simulink model "improved_z_source_inverterwithpv"  (Simulink 8.1)
settings: Solver=ode45  StartTime=0.0  StopTime=0.1  MaxStep=1e-6  RelTol=1e-3
libraries: powerlib x128, powerlib_extras x3, simulink x1
settings Model: Creator=Kashif  LastModifiedBy=Rama Krishna Reddy
settings DataIOCC: InspectSignalLogs=on
settings DebuggingCC: SaveWithParameterizedLinksMsg=none  StrictBusMsg=Warning

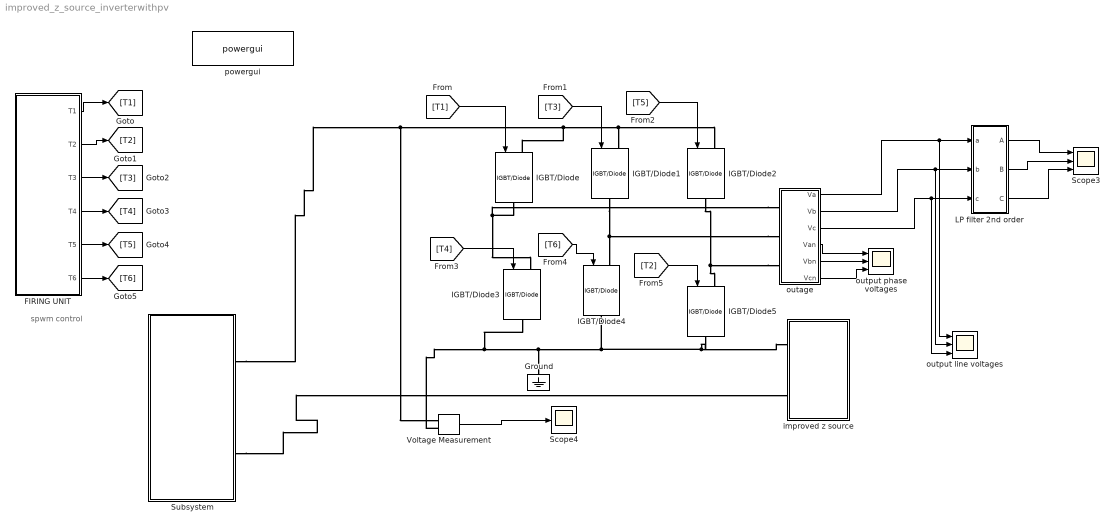
== system improved_z_source_inverterwithpv ==
  note: spwm control
  FIRING UNIT : Subsystem
  Ground : powerlib/Elements/Ground  LConnTagsString=a
  IGBT/Diode{,1..5} (6 alike) : powerlib/Power Electronics/IGBT//Diode  Ron=1e-3  Rs=1e5  Cs=inf  Measurements=off
  LP filter 2nd order : Subsystem  mask{cutoff_frequency=100, damping_factor=0.707}
      mask prompts: cutoff_frequency "Cut off frequency"; damping_factor "Damping Factor"
  Scope3 : Scope  NumInputPorts=3
      settings: TickLabels=on  YMin=-400~-400~-400  YMax=400~400~400  SaveName=Filtered_voltages  MaxDataPoints=5000000  SampleInput=on  SampleTime=5e-6
  Scope4 : Scope
      settings: YMin=362.27  YMax=362.37  SaveName=Neutral_voltages1  MaxDataPoints=5000000  SampleInput=on  SampleTime=5e-6
  Subsystem : Subsystem
  Voltage Measurement : powerlib/Measurements/Voltage Measurement  PhasorSimulation=off  OutputType=Complex  PSBequivalent=0
  improved z source : Subsystem
  outage : Subsystem
  output line voltages : Scope  NumInputPorts=3
      settings: YMin=-5~-5~-5  YMax=5~5~5  SaveName=Line_voltages  MaxDataPoints=5000000  SampleInput=on  SampleTime=5e-6
  output phase voltages : Scope  NumInputPorts=3
      settings: YMin=-250~-250~-250  YMax=250~250~250  SaveName=Neutral_voltages  MaxDataPoints=5000000  SampleInput=on  SampleTime=5e-6
  powergui : powerlib/powergui  Priority=1  SimulationMode=Discrete  SolverType=Tustin  SampleTime=5e-6  frequency=60  SPID=off  DisableSnubberDevices=off  DisableRonSwitches=off  DisableVfSwitches=off  SwTol=0  Interpol=off  DisplayEquations=off  frequencyindice=0  Pbase=100e6  ErrMax=1e-4  Iterations=50  UnitsV=kV  UnitsW=MW  FunctionMessages=off  echomessages=off  HookPort=off  EnableUseOfTLC=off  x0status=blocks  RestoreLinks=warning  ResistiveCurrentMeasurement=off  Frange=[0:2:500]  Ylog=off  Xlog=on  ShowGrid=off  save=off  variable=ZData  structure=Neutral_voltages  ZoomFFT=off  StartTime=0.04  cycles=3  DisplayStyle=2  fundamental=50  FreqAxis=off  MaxFrequency=1000  frequencyindicesteady=1  RmsSteady=1  display=off  Ts=0  methode=off
  wires:
  outage/2(Vb) -> output line voltages/2, LP filter 2nd order/2(b)
  outage/3(Vc) -> output line voltages/3, LP filter 2nd order/3(c)
  outage/4(Van) -> output phase voltages/1
  outage/5(Vbn) -> output phase voltages/2
  outage/6(Vcn) -> output phase voltages/3
  [T3] -> IGBT/Diode1/1
  [T5] -> IGBT/Diode2/1
  [T4] -> IGBT/Diode3/1
  [T6] -> IGBT/Diode4/1
  [T2] -> IGBT/Diode5/1
  [T1] -> IGBT/Diode/1
  FIRING UNIT/1(T1) -> [T1]
  FIRING UNIT/2(T2) -> [T2]
  FIRING UNIT/3(T3) -> [T3]
  FIRING UNIT/4(T4) -> [T4]
  FIRING UNIT/5(T5) -> [T5]
  FIRING UNIT/6(T6) -> [T6]
  outage/1(Va) -> output line voltages/1, LP filter 2nd order/1(a)
  LP filter 2nd order/3(C) -> Scope3/3
  LP filter 2nd order/2(B) -> Scope3/2
  LP filter 2nd order/1(A) -> Scope3/1
  Voltage Measurement/1 -> Scope4/1
  connections:
  outage/LConn1 -- IGBT/Diode3/LConn1 -- IGBT/Diode/RConn1
  outage/LConn2 -- IGBT/Diode4/LConn1 -- IGBT/Diode1/RConn1
  outage/LConn3 -- IGBT/Diode2/RConn1 -- IGBT/Diode5/LConn1
  Voltage Measurement/LConn2 -- IGBT/Diode4/RConn1 -- IGBT/Diode5/RConn1 -- improved z source/LConn1 -- Ground/LConn1 -- IGBT/Diode3/RConn1
  Subsystem/RConn1 -- IGBT/Diode1/LConn1 -- IGBT/Diode2/LConn1 -- IGBT/Diode/LConn1 -- Voltage Measurement/LConn1
  Subsystem/RConn2 -- improved z source/LConn2

== system improved_z_source_inverterwithpv/FIRING UNIT ==
  note: 3-phase input
  Subsystem2 : Subsystem
  Subsystem3 : Subsystem
  T1 : Outport
  T2 : Outport  Port=2
  T3 : Outport  Port=3
  T4 : Outport  Port=4
  T5 : Outport  Port=5
  T6 : Outport  Port=6
  wires:
  Subsystem2/3(SinewaveC) -> Subsystem3/3(In3)
  Subsystem3/1(A1) -> T1/1
  Subsystem3/2(C2) -> T2/1
  Subsystem3/3(B1) -> T3/1
  Subsystem3/4(A2) -> T4/1
  Subsystem3/5(B2) -> T6/1
  Subsystem3/6(C1) -> T5/1
  Subsystem2/1(SinewaveA) -> Subsystem3/1(In1)
  Subsystem2/2(SinewaveB) -> Subsystem3/2(In2)

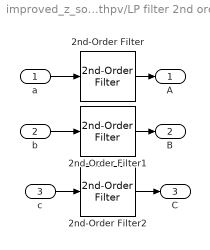
== system improved_z_source_inverterwithpv/LP filter 2nd order ==
  a : Inport
  b : Inport  Port=2
  c : Inport  Port=3
  2nd-Order Filter : powerlib_extras/Control  Blocks/2nd-Order Filter  FilterType=Lowpass  Fo=cutoff_frequency  Zeta=damping_factor  Initialize=off  Vac_Init=[1 45 60]  Vdc_Init=-0.5  PlotResponse=off  param1=[1 500 1]
  2nd-Order Filter1 : powerlib_extras/Control  Blocks/2nd-Order Filter  FilterType=Lowpass  Fo=cutoff_frequency  Zeta=damping_factor  Initialize=off  Vac_Init=[1 45 60]  Vdc_Init=-0.5  PlotResponse=off  param1=[1 500 1]
  2nd-Order Filter2 : powerlib_extras/Control  Blocks/2nd-Order Filter  FilterType=Lowpass  Fo=cutoff_frequency  Zeta=damping_factor  Initialize=off  Vac_Init=[1 45 60]  Vdc_Init=-0.5  PlotResponse=off  param1=[1 500 1]
  A : Outport
  B : Outport  Port=2
  C : Outport  Port=3
  wires:
  a/1 -> 2nd-Order Filter/1
  2nd-Order Filter/1 -> A/1
  b/1 -> 2nd-Order Filter1/1
  2nd-Order Filter1/1 -> B/1
  c/1 -> 2nd-Order Filter2/1
  2nd-Order Filter2/1 -> C/1

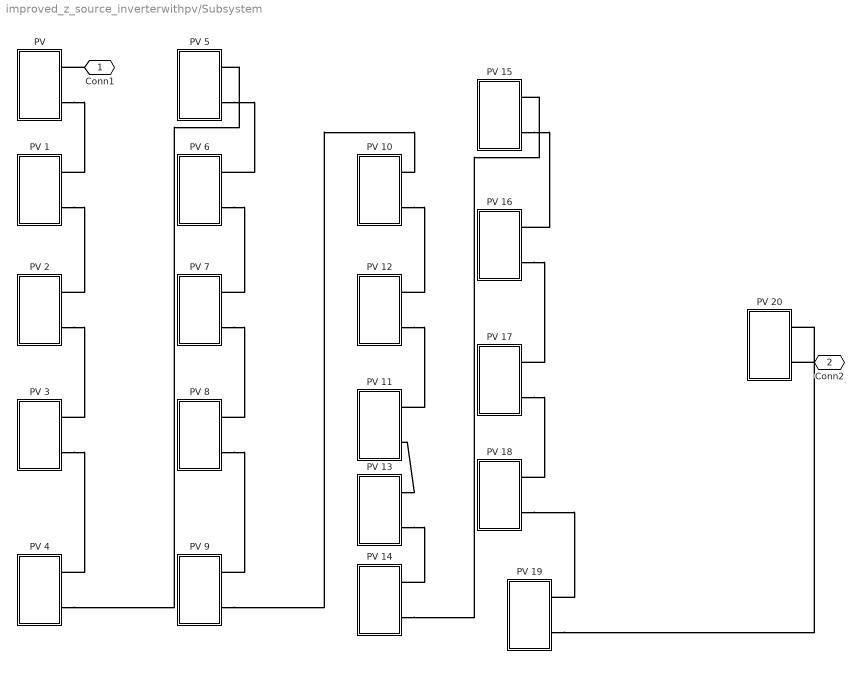
== system improved_z_source_inverterwithpv/Subsystem ==
  "PV " : Subsystem
  PV 1 : Subsystem
  PV 10 : Subsystem
  PV 11 : Subsystem
  PV 12 : Subsystem
  PV 13 : Subsystem
  PV 14 : Subsystem
  PV 15 : Subsystem
  PV 16 : Subsystem
  PV 17 : Subsystem
  PV 18 : Subsystem
  PV 19 : Subsystem
  PV 2 : Subsystem
  PV 20 : Subsystem
  PV 3 : Subsystem
  PV 4 : Subsystem
  PV 5 : Subsystem
  PV 6 : Subsystem
  PV 7 : Subsystem
  PV 8 : Subsystem
  PV 9 : Subsystem
  Conn1 : PMIOPort  Port=1  Side=Right
  Conn2 : PMIOPort  Port=2  Side=Right
  connections:
  "PV "/RConn2 -- PV 1/RConn1
  PV 1/RConn2 -- PV 2/RConn1
  PV 9/RConn2 -- PV 10/RConn1
  PV 10/RConn2 -- PV 12/RConn1
  PV 12/RConn2 -- PV 11/RConn1
  PV 13/RConn1 -- PV 11/RConn2
  PV 13/RConn2 -- PV 14/RConn1
  PV 14/RConn2 -- PV 15/RConn1
  PV 15/RConn2 -- PV 16/RConn1
  PV 16/RConn2 -- PV 17/RConn1
  PV 17/RConn2 -- PV 18/RConn1
  PV 18/RConn2 -- PV 19/RConn1
  PV 19/RConn2 -- PV 20/RConn1
  PV 2/RConn2 -- PV 3/RConn1
  PV 3/RConn2 -- PV 4/RConn1
  PV 4/RConn2 -- PV 5/RConn1
  PV 5/RConn2 -- PV 6/RConn1
  PV 6/RConn2 -- PV 7/RConn1
  PV 7/RConn2 -- PV 8/RConn1
  PV 8/RConn2 -- PV 9/RConn1
  Conn1/RConn1 -- "PV "/RConn1
  Conn2/RConn1 -- PV 20/RConn2

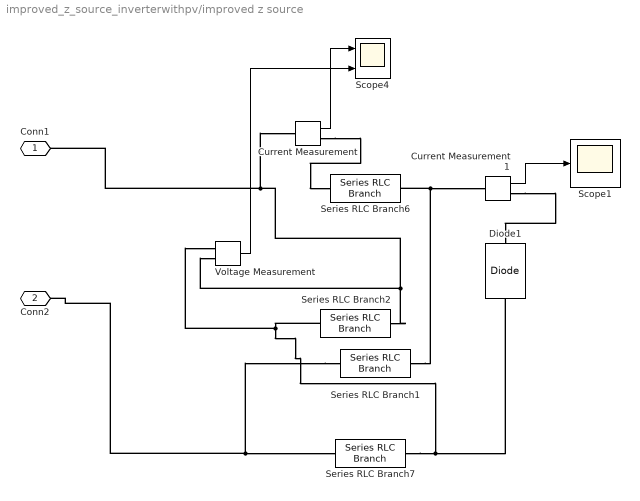
== system improved_z_source_inverterwithpv/improved z source ==
  Current Measurement : powerlib/Measurements/Current Measurement  PhasorSimulation=off  OutputType=Complex  PSBequivalent=0
  Current Measurement1 : powerlib/Measurements/Current Measurement  PhasorSimulation=off  OutputType=Complex  PSBequivalent=0
  Diode1 : powerlib/Power Electronics/Diode  Ron=0.001  Lon=0  Vf=0.8  IC=0  UseSnubber=off  Rs=500  Cs=250e-9  Measurements=off
  Scope1 : Scope
      settings: YMin=6.7775e-007  YMax=6.815e-007  SaveName=Line_voltages2  MaxDataPoints=5000000  SampleInput=on  SampleTime=5e-6
  Scope4 : Scope  NumInputPorts=2
      settings: YMin=-5~-5  YMax=5~5
  Series RLC Branch1 : powerlib/Elements/Series RLC Branch  LConnTagsString=__new0  RConnTagsString=__new0  BranchType=C  Resistance=1  Inductance=1e-3  SetiL0=off  InitialCurrent=0  Capacitance=2000e-6  Setx0=off  InitialVoltage=0  Measurements=None
  Series RLC Branch2 : powerlib/Elements/Series RLC Branch  LConnTagsString=__new0  RConnTagsString=__new0  BranchType=C  Resistance=1  Inductance=1e-3  SetiL0=off  InitialCurrent=0  Capacitance=2000e-6  Setx0=off  InitialVoltage=0  Measurements=None
  Series RLC Branch6 : powerlib/Elements/Series RLC Branch  LConnTagsString=__new0  RConnTagsString=__new0  BranchType=L  Resistance=1  Inductance=1000e-6  SetiL0=off  InitialCurrent=0  Capacitance=1e-6  Setx0=off  InitialVoltage=0  Measurements=None
  Series RLC Branch7 : powerlib/Elements/Series RLC Branch  LConnTagsString=__new0  RConnTagsString=__new0  BranchType=L  Resistance=1  Inductance=1000e-6  SetiL0=off  InitialCurrent=0  Capacitance=1e-6  Setx0=off  InitialVoltage=0  Measurements=None
  Voltage Measurement : powerlib/Measurements/Voltage Measurement  PhasorSimulation=off  OutputType=Complex  PSBequivalent=0
  Conn1 : PMIOPort  Port=1  Side=Left
  Conn2 : PMIOPort  Port=2  Side=Left
  wires:
  Current Measurement/1 -> Scope4/1
  Voltage Measurement/1 -> Scope4/2
  Current Measurement1/1 -> Scope1/1
  connections:
  Series RLC Branch2/RConn1 -- Current Measurement/LConn1 -- Conn1/RConn1 -- Voltage Measurement/LConn2
  Current Measurement/RConn1 -- Series RLC Branch6/LConn1
  Series RLC Branch1/RConn1 -- Series RLC Branch6/RConn1 -- Current Measurement1/LConn1
  Series RLC Branch2/LConn1 -- Diode1/RConn1 -- Series RLC Branch7/RConn1 -- Voltage Measurement/LConn1
  Series RLC Branch1/LConn1 -- Series RLC Branch7/LConn1 -- Conn2/RConn1
  Current Measurement1/RConn1 -- Diode1/LConn1

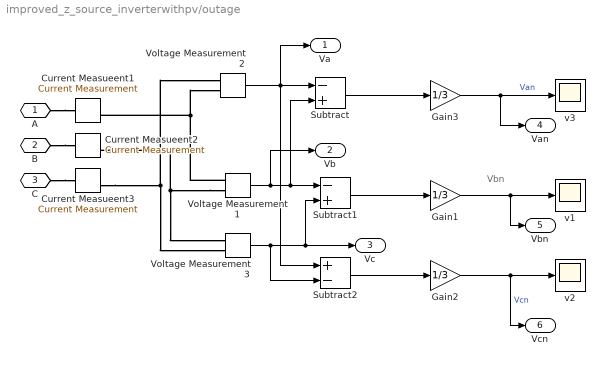
== system improved_z_source_inverterwithpv/outage ==
  note: Vbn
  Current Measueent1 : powerlib/Measurements/Current Measurement  PhasorSimulation=off  OutputType=Complex  PSBequivalent=0
  Current Measueent2 : powerlib/Measurements/Current Measurement  PhasorSimulation=off  OutputType=Complex  PSBequivalent=0
  Current Measueent3 : powerlib/Measurements/Current Measurement  PhasorSimulation=off  OutputType=Complex  PSBequivalent=0
  Gain1 : Gain  Gain=1/3
  Gain2 : Gain  Gain=1/3
  Gain3 : Gain  Gain=1/3
  Subtract : Sum  Inputs=-+
  Subtract1 : Sum  Inputs=-+
  Subtract2 : Sum  Inputs=+-
  Voltage Measurement1 : powerlib/Measurements/Voltage Measurement  PhasorSimulation=off  OutputType=Complex  PSBequivalent=0
  Voltage Measurement2 : powerlib/Measurements/Voltage Measurement  PhasorSimulation=off  OutputType=Complex  PSBequivalent=0
  Voltage Measurement3 : powerlib/Measurements/Voltage Measurement  PhasorSimulation=off  OutputType=Complex  PSBequivalent=0
  v1 : Scope
      settings: SaveName=ScopeData25  MaxDataPoints=5000000
  v2 : Scope
      settings: SaveName=ScopeData26  MaxDataPoints=5000000
  v3 : Scope
      settings: YMin=-300  YMax=300  SaveName=ScopeData27  MaxDataPoints=5000000
  A : PMIOPort  Port=1  Side=Left
  B : PMIOPort  Port=2  Side=Left
  C : PMIOPort  Port=3  Side=Left
  Va : Outport
  Vb : Outport  Port=2
  Vc : Outport  Port=3
  Van : Outport  Port=4
  Vbn : Outport  Port=5
  Vcn : Outport  Port=6
  wires:
  Gain2/1 -> v2/1, Vcn/1  "Vcn"
  Subtract2/1 -> Gain2/1
  Gain1/1 -> v1/1, Vbn/1
  Subtract1/1 -> Gain1/1
  Voltage Measurement3/1 -> Subtract2/2, Subtract1/2, Vc/1
  Gain3/1 -> v3/1, Van/1  "Van"
  Subtract/1 -> Gain3/1
  Voltage Measurement1/1 -> Subtract/2, Subtract1/1, Vb/1
  Voltage Measurement2/1 -> Subtract/1, Subtract2/1, Va/1
  connections:
  Voltage Measurement1/LConn1 -- Current Measueent1/RConn1 -- Voltage Measurement2/LConn2
  Voltage Measurement1/LConn2 -- Current Measueent2/RConn1 -- Voltage Measurement3/LConn1
  Current Measueent3/RConn1 -- Voltage Measurement2/LConn1 -- Voltage Measurement3/LConn2
  A/RConn1 -- Current Measueent1/LConn1
  B/RConn1 -- Current Measueent2/LConn1
  C/RConn1 -- Current Measueent3/LConn1

== system improved_z_source_inverterwithpv/FIRING UNIT/Subsystem2 ==
  V_control,A : Sin  Amplitude=8  Frequency=50*2*pi  SampleTime=0
  V_control,B : Sin  Amplitude=8  Frequency=50*2*pi  Phase=2*pi/3  SampleTime=0
  V_control,C : Sin  Amplitude=8  Frequency=50*2*pi  Phase=4*pi/3  SampleTime=0
  SinewaveA : Outport
  SinewaveB : Outport  Port=2
  SinewaveC : Outport  Port=3
  wires:
  V_control,A/1 -> SinewaveA/1
  V_control,B/1 -> SinewaveB/1
  V_control,C/1 -> SinewaveC/1

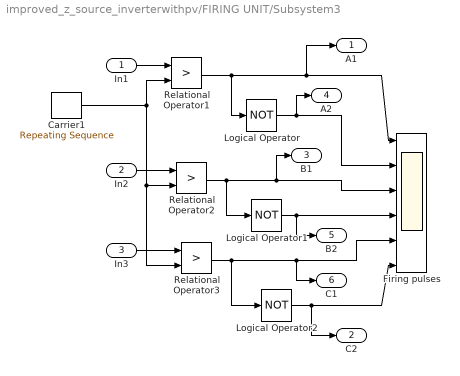
== system improved_z_source_inverterwithpv/FIRING UNIT/Subsystem3 ==
  In1 : Inport
  In2 : Inport  Port=2
  In3 : Inport  Port=3
  Carrier1 : simulink/Sources/Repeating Sequence  rep_seq_t="[0 (1/20000)/4 (1/20000)*3/4  1/20000]"  rep_seq_y=[0 6 -6 0]
  Firing pulses : Scope  NumInputPorts=6
      settings: YMin=0~0~-1~0~0~0  YMax=1~1~1~2~1~1
  Logical Operator : Logic  Operator=NOT
  Logical Operator1 : Logic  Operator=NOT
  Logical Operator2 : Logic  Operator=NOT
  Relational Operator1 : RelationalOperator  Operator=>  InputSameDT=on
  Relational Operator2 : RelationalOperator  Operator=>  InputSameDT=on
  Relational Operator3 : RelationalOperator  Operator=>  InputSameDT=on
  A1 : Outport
  C2 : Outport  Port=2
  B1 : Outport  Port=3
  A2 : Outport  Port=4
  B2 : Outport  Port=5
  C1 : Outport  Port=6
  wires:
  Relational Operator1/1 -> Logical Operator/1, Firing pulses/1, A1/1
  Relational Operator2/1 -> Logical Operator1/1, Firing pulses/3, B1/1
  Relational Operator3/1 -> Logical Operator2/1, Firing pulses/5, C1/1
  Logical Operator/1 -> Firing pulses/2, A2/1
  Logical Operator1/1 -> Firing pulses/4, B2/1
  Logical Operator2/1 -> Firing pulses/6, C2/1
  Carrier1/1 -> Relational Operator2/2, Relational Operator3/2, Relational Operator1/2
  In1/1 -> Relational Operator1/1
  In2/1 -> Relational Operator2/1
  In3/1 -> Relational Operator3/1

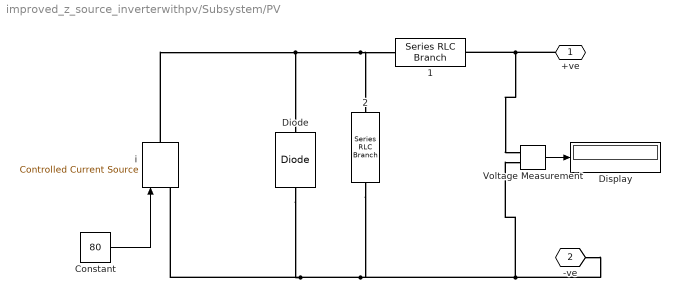
== system improved_z_source_inverterwithpv/Subsystem/PV  ==
  1 : powerlib/Elements/Series RLC Branch  LConnTagsString=__new0  RConnTagsString=__new0  BranchType=R  Resistance=0.001  Inductance=1e-3  SetiL0=off  InitialCurrent=0  Capacitance=1e-6  Setx0=off  InitialVoltage=0  Measurements=None
  2 : powerlib/Elements/Series RLC Branch  LConnTagsString=__new0  RConnTagsString=__new0  BranchType=R  Resistance=10000  Inductance=1e-3  SetiL0=off  InitialCurrent=0  Capacitance=1e-6  Setx0=off  InitialVoltage=0  Measurements=None
  Constant : Constant  Value=80
  Diode : powerlib/Power Electronics/Diode  Ron=0.001  Lon=0  Vf=20  IC=0  UseSnubber=off  Rs=500  Cs=250e-9  Measurements=off
  Display : Display
  Voltage Measurement : powerlib/Measurements/Voltage Measurement  PhasorSimulation=off  OutputType=Complex  PSBequivalent=0
  i : powerlib/Electrical Sources/Controlled Current Source  Initialize=on  Source_Type=AC  Amplitude=0  Phase=0  Frequency=0  Measurements=None
  +ve : PMIOPort  Port=1  Side=Right
  -ve : PMIOPort  Tag=PMCPort  Port=2  Side=Right
  wires:
  Constant/1 -> i/1
  Voltage Measurement/1 -> Display/1
  connections:
  i/RConn1 -- Diode/LConn1 -- 1/LConn1 -- 2/LConn1
  i/LConn1 -- Diode/RConn1 -- 2/RConn1 -- -ve/RConn1 -- Voltage Measurement/LConn2
  +ve/RConn1 -- 1/RConn1 -- Voltage Measurement/LConn1

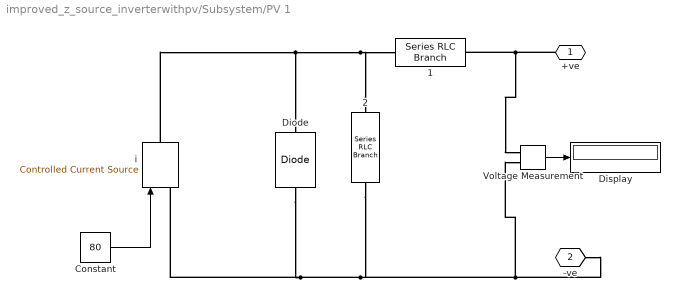
== system improved_z_source_inverterwithpv/Subsystem/PV 1 ==
  1 : powerlib/Elements/Series RLC Branch  LConnTagsString=__new0  RConnTagsString=__new0  BranchType=R  Resistance=0.001  Inductance=1e-3  SetiL0=off  InitialCurrent=0  Capacitance=1e-6  Setx0=off  InitialVoltage=0  Measurements=None
  2 : powerlib/Elements/Series RLC Branch  LConnTagsString=__new0  RConnTagsString=__new0  BranchType=R  Resistance=10000  Inductance=1e-3  SetiL0=off  InitialCurrent=0  Capacitance=1e-6  Setx0=off  InitialVoltage=0  Measurements=None
  Constant : Constant  Value=80
  Diode : powerlib/Power Electronics/Diode  Ron=0.001  Lon=0  Vf=20  IC=0  UseSnubber=off  Rs=500  Cs=250e-9  Measurements=off
  Display : Display
  Voltage Measurement : powerlib/Measurements/Voltage Measurement  PhasorSimulation=off  OutputType=Complex  PSBequivalent=0
  i : powerlib/Electrical Sources/Controlled Current Source  Initialize=on  Source_Type=AC  Amplitude=0  Phase=0  Frequency=0  Measurements=None
  +ve : PMIOPort  Port=1  Side=Right
  -ve : PMIOPort  Tag=PMCPort  Port=2  Side=Right
  wires:
  Voltage Measurement/1 -> Display/1
  Constant/1 -> i/1
  connections:
  Voltage Measurement/LConn1 -- 1/RConn1 -- +ve/RConn1
  Voltage Measurement/LConn2 -- -ve/RConn1 -- 2/RConn1 -- Diode/RConn1 -- i/LConn1
  2/LConn1 -- 1/LConn1 -- Diode/LConn1 -- i/RConn1

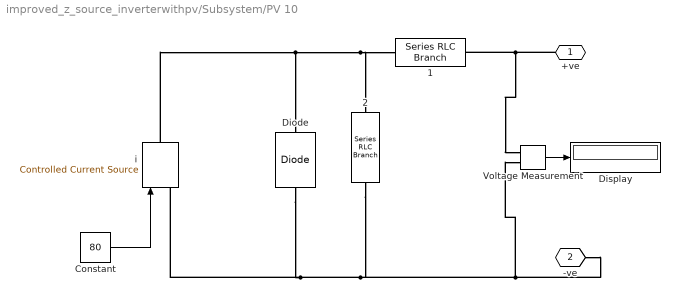
== system improved_z_source_inverterwithpv/Subsystem/PV 10 ==
  1 : powerlib/Elements/Series RLC Branch  LConnTagsString=__new0  RConnTagsString=__new0  BranchType=R  Resistance=0.001  Inductance=1e-3  SetiL0=off  InitialCurrent=0  Capacitance=1e-6  Setx0=off  InitialVoltage=0  Measurements=None
  2 : powerlib/Elements/Series RLC Branch  LConnTagsString=__new0  RConnTagsString=__new0  BranchType=R  Resistance=10000  Inductance=1e-3  SetiL0=off  InitialCurrent=0  Capacitance=1e-6  Setx0=off  InitialVoltage=0  Measurements=None
  Constant : Constant  Value=80
  Diode : powerlib/Power Electronics/Diode  Ron=0.001  Lon=0  Vf=20  IC=0  UseSnubber=off  Rs=500  Cs=250e-9  Measurements=off
  Display : Display
  Voltage Measurement : powerlib/Measurements/Voltage Measurement  PhasorSimulation=off  OutputType=Complex  PSBequivalent=0
  i : powerlib/Electrical Sources/Controlled Current Source  Initialize=on  Source_Type=AC  Amplitude=0  Phase=0  Frequency=0  Measurements=None
  +ve : PMIOPort  Port=1  Side=Right
  -ve : PMIOPort  Tag=PMCPort  Port=2  Side=Right
  wires:
  Constant/1 -> i/1
  Voltage Measurement/1 -> Display/1
  connections:
  i/RConn1 -- Diode/LConn1 -- 1/LConn1 -- 2/LConn1
  i/LConn1 -- Diode/RConn1 -- 2/RConn1 -- -ve/RConn1 -- Voltage Measurement/LConn2
  +ve/RConn1 -- 1/RConn1 -- Voltage Measurement/LConn1

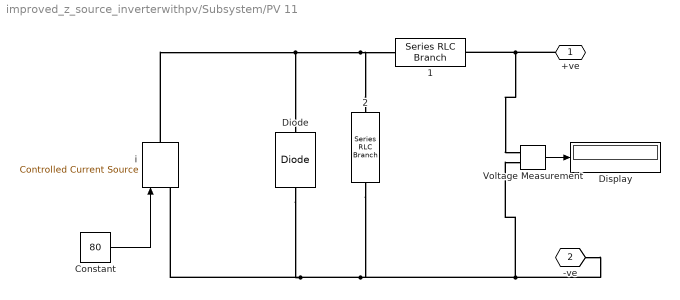
== system improved_z_source_inverterwithpv/Subsystem/PV 11 ==
  1 : powerlib/Elements/Series RLC Branch  LConnTagsString=__new0  RConnTagsString=__new0  BranchType=R  Resistance=0.001  Inductance=1e-3  SetiL0=off  InitialCurrent=0  Capacitance=1e-6  Setx0=off  InitialVoltage=0  Measurements=None
  2 : powerlib/Elements/Series RLC Branch  LConnTagsString=__new0  RConnTagsString=__new0  BranchType=R  Resistance=10000  Inductance=1e-3  SetiL0=off  InitialCurrent=0  Capacitance=1e-6  Setx0=off  InitialVoltage=0  Measurements=None
  Constant : Constant  Value=80
  Diode : powerlib/Power Electronics/Diode  Ron=0.001  Lon=0  Vf=20  IC=0  UseSnubber=off  Rs=500  Cs=250e-9  Measurements=off
  Display : Display
  Voltage Measurement : powerlib/Measurements/Voltage Measurement  PhasorSimulation=off  OutputType=Complex  PSBequivalent=0
  i : powerlib/Electrical Sources/Controlled Current Source  Initialize=on  Source_Type=AC  Amplitude=0  Phase=0  Frequency=0  Measurements=None
  +ve : PMIOPort  Port=1  Side=Right
  -ve : PMIOPort  Tag=PMCPort  Port=2  Side=Right
  wires:
  Voltage Measurement/1 -> Display/1
  Constant/1 -> i/1
  connections:
  Voltage Measurement/LConn1 -- 1/RConn1 -- +ve/RConn1
  Voltage Measurement/LConn2 -- -ve/RConn1 -- 2/RConn1 -- Diode/RConn1 -- i/LConn1
  2/LConn1 -- 1/LConn1 -- Diode/LConn1 -- i/RConn1

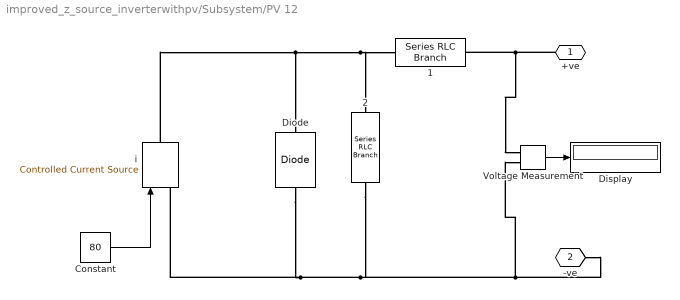
== system improved_z_source_inverterwithpv/Subsystem/PV 12 ==
  1 : powerlib/Elements/Series RLC Branch  LConnTagsString=__new0  RConnTagsString=__new0  BranchType=R  Resistance=0.001  Inductance=1e-3  SetiL0=off  InitialCurrent=0  Capacitance=1e-6  Setx0=off  InitialVoltage=0  Measurements=None
  2 : powerlib/Elements/Series RLC Branch  LConnTagsString=__new0  RConnTagsString=__new0  BranchType=R  Resistance=10000  Inductance=1e-3  SetiL0=off  InitialCurrent=0  Capacitance=1e-6  Setx0=off  InitialVoltage=0  Measurements=None
  Constant : Constant  Value=80
  Diode : powerlib/Power Electronics/Diode  Ron=0.001  Lon=0  Vf=20  IC=0  UseSnubber=off  Rs=500  Cs=250e-9  Measurements=off
  Display : Display
  Voltage Measurement : powerlib/Measurements/Voltage Measurement  PhasorSimulation=off  OutputType=Complex  PSBequivalent=0
  i : powerlib/Electrical Sources/Controlled Current Source  Initialize=on  Source_Type=AC  Amplitude=0  Phase=0  Frequency=0  Measurements=None
  +ve : PMIOPort  Port=1  Side=Right
  -ve : PMIOPort  Tag=PMCPort  Port=2  Side=Right
  wires:
  Constant/1 -> i/1
  Voltage Measurement/1 -> Display/1
  connections:
  i/RConn1 -- Diode/LConn1 -- 1/LConn1 -- 2/LConn1
  i/LConn1 -- Diode/RConn1 -- 2/RConn1 -- -ve/RConn1 -- Voltage Measurement/LConn2
  +ve/RConn1 -- 1/RConn1 -- Voltage Measurement/LConn1

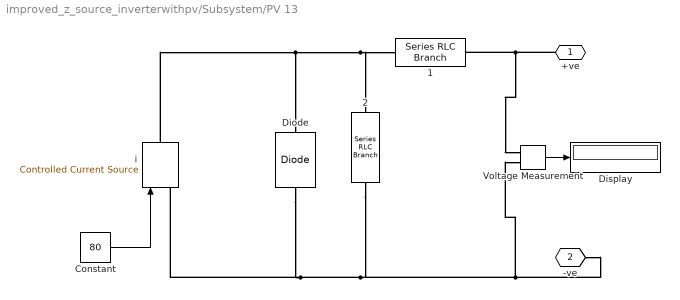
== system improved_z_source_inverterwithpv/Subsystem/PV 13 ==
  1 : powerlib/Elements/Series RLC Branch  LConnTagsString=__new0  RConnTagsString=__new0  BranchType=R  Resistance=0.001  Inductance=1e-3  SetiL0=off  InitialCurrent=0  Capacitance=1e-6  Setx0=off  InitialVoltage=0  Measurements=None
  2 : powerlib/Elements/Series RLC Branch  LConnTagsString=__new0  RConnTagsString=__new0  BranchType=R  Resistance=10000  Inductance=1e-3  SetiL0=off  InitialCurrent=0  Capacitance=1e-6  Setx0=off  InitialVoltage=0  Measurements=None
  Constant : Constant  Value=80
  Diode : powerlib/Power Electronics/Diode  Ron=0.001  Lon=0  Vf=20  IC=0  UseSnubber=off  Rs=500  Cs=250e-9  Measurements=off
  Display : Display
  Voltage Measurement : powerlib/Measurements/Voltage Measurement  PhasorSimulation=off  OutputType=Complex  PSBequivalent=0
  i : powerlib/Electrical Sources/Controlled Current Source  Initialize=on  Source_Type=AC  Amplitude=0  Phase=0  Frequency=0  Measurements=None
  +ve : PMIOPort  Port=1  Side=Right
  -ve : PMIOPort  Tag=PMCPort  Port=2  Side=Right
  wires:
  Constant/1 -> i/1
  Voltage Measurement/1 -> Display/1
  connections:
  i/RConn1 -- Diode/LConn1 -- 1/LConn1 -- 2/LConn1
  i/LConn1 -- Diode/RConn1 -- 2/RConn1 -- -ve/RConn1 -- Voltage Measurement/LConn2
  +ve/RConn1 -- 1/RConn1 -- Voltage Measurement/LConn1

== system improved_z_source_inverterwithpv/Subsystem/PV 14 ==
  1 : powerlib/Elements/Series RLC Branch  LConnTagsString=__new0  RConnTagsString=__new0  BranchType=R  Resistance=0.001  Inductance=1e-3  SetiL0=off  InitialCurrent=0  Capacitance=1e-6  Setx0=off  InitialVoltage=0  Measurements=None
  2 : powerlib/Elements/Series RLC Branch  LConnTagsString=__new0  RConnTagsString=__new0  BranchType=R  Resistance=10000  Inductance=1e-3  SetiL0=off  InitialCurrent=0  Capacitance=1e-6  Setx0=off  InitialVoltage=0  Measurements=None
  Constant : Constant  Value=80
  Diode : powerlib/Power Electronics/Diode  Ron=0.001  Lon=0  Vf=20  IC=0  UseSnubber=off  Rs=500  Cs=250e-9  Measurements=off
  Display : Display
  Voltage Measurement : powerlib/Measurements/Voltage Measurement  PhasorSimulation=off  OutputType=Complex  PSBequivalent=0
  i : powerlib/Electrical Sources/Controlled Current Source  Initialize=on  Source_Type=AC  Amplitude=0  Phase=0  Frequency=0  Measurements=None
  +ve : PMIOPort  Port=1  Side=Right
  -ve : PMIOPort  Tag=PMCPort  Port=2  Side=Right
  wires:
  Voltage Measurement/1 -> Display/1
  Constant/1 -> i/1
  connections:
  Voltage Measurement/LConn1 -- 1/RConn1 -- +ve/RConn1
  Voltage Measurement/LConn2 -- -ve/RConn1 -- 2/RConn1 -- Diode/RConn1 -- i/LConn1
  2/LConn1 -- 1/LConn1 -- Diode/LConn1 -- i/RConn1

== system improved_z_source_inverterwithpv/Subsystem/PV 15 ==
  1 : powerlib/Elements/Series RLC Branch  LConnTagsString=__new0  RConnTagsString=__new0  BranchType=R  Resistance=0.001  Inductance=1e-3  SetiL0=off  InitialCurrent=0  Capacitance=1e-6  Setx0=off  InitialVoltage=0  Measurements=None
  2 : powerlib/Elements/Series RLC Branch  LConnTagsString=__new0  RConnTagsString=__new0  BranchType=R  Resistance=10000  Inductance=1e-3  SetiL0=off  InitialCurrent=0  Capacitance=1e-6  Setx0=off  InitialVoltage=0  Measurements=None
  Constant : Constant  Value=80
  Diode : powerlib/Power Electronics/Diode  Ron=0.001  Lon=0  Vf=20  IC=0  UseSnubber=off  Rs=500  Cs=250e-9  Measurements=off
  Display : Display
  Voltage Measurement : powerlib/Measurements/Voltage Measurement  PhasorSimulation=off  OutputType=Complex  PSBequivalent=0
  i : powerlib/Electrical Sources/Controlled Current Source  Initialize=on  Source_Type=AC  Amplitude=0  Phase=0  Frequency=0  Measurements=None
  +ve : PMIOPort  Port=1  Side=Right
  -ve : PMIOPort  Tag=PMCPort  Port=2  Side=Right
  wires:
  Voltage Measurement/1 -> Display/1
  Constant/1 -> i/1
  connections:
  Voltage Measurement/LConn1 -- 1/RConn1 -- +ve/RConn1
  Voltage Measurement/LConn2 -- -ve/RConn1 -- 2/RConn1 -- Diode/RConn1 -- i/LConn1
  2/LConn1 -- 1/LConn1 -- Diode/LConn1 -- i/RConn1

== system improved_z_source_inverterwithpv/Subsystem/PV 16 ==
  1 : powerlib/Elements/Series RLC Branch  LConnTagsString=__new0  RConnTagsString=__new0  BranchType=R  Resistance=0.001  Inductance=1e-3  SetiL0=off  InitialCurrent=0  Capacitance=1e-6  Setx0=off  InitialVoltage=0  Measurements=None
  2 : powerlib/Elements/Series RLC Branch  LConnTagsString=__new0  RConnTagsString=__new0  BranchType=R  Resistance=10000  Inductance=1e-3  SetiL0=off  InitialCurrent=0  Capacitance=1e-6  Setx0=off  InitialVoltage=0  Measurements=None
  Constant : Constant  Value=80
  Diode : powerlib/Power Electronics/Diode  Ron=0.001  Lon=0  Vf=20  IC=0  UseSnubber=off  Rs=500  Cs=250e-9  Measurements=off
  Display : Display
  Voltage Measurement : powerlib/Measurements/Voltage Measurement  PhasorSimulation=off  OutputType=Complex  PSBequivalent=0
  i : powerlib/Electrical Sources/Controlled Current Source  Initialize=on  Source_Type=AC  Amplitude=0  Phase=0  Frequency=0  Measurements=None
  +ve : PMIOPort  Port=1  Side=Right
  -ve : PMIOPort  Tag=PMCPort  Port=2  Side=Right
  wires:
  Constant/1 -> i/1
  Voltage Measurement/1 -> Display/1
  connections:
  i/RConn1 -- Diode/LConn1 -- 1/LConn1 -- 2/LConn1
  i/LConn1 -- Diode/RConn1 -- 2/RConn1 -- -ve/RConn1 -- Voltage Measurement/LConn2
  +ve/RConn1 -- 1/RConn1 -- Voltage Measurement/LConn1

== system improved_z_source_inverterwithpv/Subsystem/PV 17 ==
  1 : powerlib/Elements/Series RLC Branch  LConnTagsString=__new0  RConnTagsString=__new0  BranchType=R  Resistance=0.001  Inductance=1e-3  SetiL0=off  InitialCurrent=0  Capacitance=1e-6  Setx0=off  InitialVoltage=0  Measurements=None
  2 : powerlib/Elements/Series RLC Branch  LConnTagsString=__new0  RConnTagsString=__new0  BranchType=R  Resistance=10000  Inductance=1e-3  SetiL0=off  InitialCurrent=0  Capacitance=1e-6  Setx0=off  InitialVoltage=0  Measurements=None
  Constant : Constant  Value=80
  Diode : powerlib/Power Electronics/Diode  Ron=0.001  Lon=0  Vf=20  IC=0  UseSnubber=off  Rs=500  Cs=250e-9  Measurements=off
  Display : Display
  Voltage Measurement : powerlib/Measurements/Voltage Measurement  PhasorSimulation=off  OutputType=Complex  PSBequivalent=0
  i : powerlib/Electrical Sources/Controlled Current Source  Initialize=on  Source_Type=AC  Amplitude=0  Phase=0  Frequency=0  Measurements=None
  +ve : PMIOPort  Port=1  Side=Right
  -ve : PMIOPort  Tag=PMCPort  Port=2  Side=Right
  wires:
  Voltage Measurement/1 -> Display/1
  Constant/1 -> i/1
  connections:
  Voltage Measurement/LConn1 -- 1/RConn1 -- +ve/RConn1
  Voltage Measurement/LConn2 -- -ve/RConn1 -- 2/RConn1 -- Diode/RConn1 -- i/LConn1
  2/LConn1 -- 1/LConn1 -- Diode/LConn1 -- i/RConn1

== system improved_z_source_inverterwithpv/Subsystem/PV 18 ==
  1 : powerlib/Elements/Series RLC Branch  LConnTagsString=__new0  RConnTagsString=__new0  BranchType=R  Resistance=0.001  Inductance=1e-3  SetiL0=off  InitialCurrent=0  Capacitance=1e-6  Setx0=off  InitialVoltage=0  Measurements=None
  2 : powerlib/Elements/Series RLC Branch  LConnTagsString=__new0  RConnTagsString=__new0  BranchType=R  Resistance=10000  Inductance=1e-3  SetiL0=off  InitialCurrent=0  Capacitance=1e-6  Setx0=off  InitialVoltage=0  Measurements=None
  Constant : Constant  Value=80
  Diode : powerlib/Power Electronics/Diode  Ron=0.001  Lon=0  Vf=20  IC=0  UseSnubber=off  Rs=500  Cs=250e-9  Measurements=off
  Display : Display
  Voltage Measurement : powerlib/Measurements/Voltage Measurement  PhasorSimulation=off  OutputType=Complex  PSBequivalent=0
  i : powerlib/Electrical Sources/Controlled Current Source  Initialize=on  Source_Type=AC  Amplitude=0  Phase=0  Frequency=0  Measurements=None
  +ve : PMIOPort  Port=1  Side=Right
  -ve : PMIOPort  Tag=PMCPort  Port=2  Side=Right
  wires:
  Constant/1 -> i/1
  Voltage Measurement/1 -> Display/1
  connections:
  i/RConn1 -- Diode/LConn1 -- 1/LConn1 -- 2/LConn1
  i/LConn1 -- Diode/RConn1 -- 2/RConn1 -- -ve/RConn1 -- Voltage Measurement/LConn2
  +ve/RConn1 -- 1/RConn1 -- Voltage Measurement/LConn1

== system improved_z_source_inverterwithpv/Subsystem/PV 19 ==
  1 : powerlib/Elements/Series RLC Branch  LConnTagsString=__new0  RConnTagsString=__new0  BranchType=R  Resistance=0.001  Inductance=1e-3  SetiL0=off  InitialCurrent=0  Capacitance=1e-6  Setx0=off  InitialVoltage=0  Measurements=None
  2 : powerlib/Elements/Series RLC Branch  LConnTagsString=__new0  RConnTagsString=__new0  BranchType=R  Resistance=10000  Inductance=1e-3  SetiL0=off  InitialCurrent=0  Capacitance=1e-6  Setx0=off  InitialVoltage=0  Measurements=None
  Constant : Constant  Value=80
  Diode : powerlib/Power Electronics/Diode  Ron=0.001  Lon=0  Vf=20  IC=0  UseSnubber=off  Rs=500  Cs=250e-9  Measurements=off
  Display : Display
  Voltage Measurement : powerlib/Measurements/Voltage Measurement  PhasorSimulation=off  OutputType=Complex  PSBequivalent=0
  i : powerlib/Electrical Sources/Controlled Current Source  Initialize=on  Source_Type=AC  Amplitude=0  Phase=0  Frequency=0  Measurements=None
  +ve : PMIOPort  Port=1  Side=Right
  -ve : PMIOPort  Tag=PMCPort  Port=2  Side=Right
  wires:
  Voltage Measurement/1 -> Display/1
  Constant/1 -> i/1
  connections:
  Voltage Measurement/LConn1 -- 1/RConn1 -- +ve/RConn1
  Voltage Measurement/LConn2 -- -ve/RConn1 -- 2/RConn1 -- Diode/RConn1 -- i/LConn1
  2/LConn1 -- 1/LConn1 -- Diode/LConn1 -- i/RConn1

== system improved_z_source_inverterwithpv/Subsystem/PV 2 ==
  1 : powerlib/Elements/Series RLC Branch  LConnTagsString=__new0  RConnTagsString=__new0  BranchType=R  Resistance=0.001  Inductance=1e-3  SetiL0=off  InitialCurrent=0  Capacitance=1e-6  Setx0=off  InitialVoltage=0  Measurements=None
  2 : powerlib/Elements/Series RLC Branch  LConnTagsString=__new0  RConnTagsString=__new0  BranchType=R  Resistance=10000  Inductance=1e-3  SetiL0=off  InitialCurrent=0  Capacitance=1e-6  Setx0=off  InitialVoltage=0  Measurements=None
  Constant : Constant  Value=80
  Diode : powerlib/Power Electronics/Diode  Ron=0.001  Lon=0  Vf=20  IC=0  UseSnubber=off  Rs=500  Cs=250e-9  Measurements=off
  Display : Display
  Voltage Measurement : powerlib/Measurements/Voltage Measurement  PhasorSimulation=off  OutputType=Complex  PSBequivalent=0
  i : powerlib/Electrical Sources/Controlled Current Source  Initialize=on  Source_Type=AC  Amplitude=0  Phase=0  Frequency=0  Measurements=None
  +ve : PMIOPort  Port=1  Side=Right
  -ve : PMIOPort  Tag=PMCPort  Port=2  Side=Right
  wires:
  Constant/1 -> i/1
  Voltage Measurement/1 -> Display/1
  connections:
  i/RConn1 -- Diode/LConn1 -- 1/LConn1 -- 2/LConn1
  i/LConn1 -- Diode/RConn1 -- 2/RConn1 -- -ve/RConn1 -- Voltage Measurement/LConn2
  +ve/RConn1 -- 1/RConn1 -- Voltage Measurement/LConn1

== system improved_z_source_inverterwithpv/Subsystem/PV 20 ==
  1 : powerlib/Elements/Series RLC Branch  LConnTagsString=__new0  RConnTagsString=__new0  BranchType=R  Resistance=0.001  Inductance=1e-3  SetiL0=off  InitialCurrent=0  Capacitance=1e-6  Setx0=off  InitialVoltage=0  Measurements=None
  2 : powerlib/Elements/Series RLC Branch  LConnTagsString=__new0  RConnTagsString=__new0  BranchType=R  Resistance=10000  Inductance=1e-3  SetiL0=off  InitialCurrent=0  Capacitance=1e-6  Setx0=off  InitialVoltage=0  Measurements=None
  Constant : Constant  Value=80
  Diode : powerlib/Power Electronics/Diode  Ron=0.001  Lon=0  Vf=20  IC=0  UseSnubber=off  Rs=500  Cs=250e-9  Measurements=off
  Display : Display
  Voltage Measurement : powerlib/Measurements/Voltage Measurement  PhasorSimulation=off  OutputType=Complex  PSBequivalent=0
  i : powerlib/Electrical Sources/Controlled Current Source  Initialize=on  Source_Type=AC  Amplitude=0  Phase=0  Frequency=0  Measurements=None
  +ve : PMIOPort  Port=1  Side=Right
  -ve : PMIOPort  Tag=PMCPort  Port=2  Side=Right
  wires:
  Constant/1 -> i/1
  Voltage Measurement/1 -> Display/1
  connections:
  i/RConn1 -- Diode/LConn1 -- 1/LConn1 -- 2/LConn1
  i/LConn1 -- Diode/RConn1 -- 2/RConn1 -- -ve/RConn1 -- Voltage Measurement/LConn2
  +ve/RConn1 -- 1/RConn1 -- Voltage Measurement/LConn1

== system improved_z_source_inverterwithpv/Subsystem/PV 3 ==
  1 : powerlib/Elements/Series RLC Branch  LConnTagsString=__new0  RConnTagsString=__new0  BranchType=R  Resistance=0.001  Inductance=1e-3  SetiL0=off  InitialCurrent=0  Capacitance=1e-6  Setx0=off  InitialVoltage=0  Measurements=None
  2 : powerlib/Elements/Series RLC Branch  LConnTagsString=__new0  RConnTagsString=__new0  BranchType=R  Resistance=10000  Inductance=1e-3  SetiL0=off  InitialCurrent=0  Capacitance=1e-6  Setx0=off  InitialVoltage=0  Measurements=None
  Constant : Constant  Value=80
  Diode : powerlib/Power Electronics/Diode  Ron=0.001  Lon=0  Vf=20  IC=0  UseSnubber=off  Rs=500  Cs=250e-9  Measurements=off
  Display : Display
  Voltage Measurement : powerlib/Measurements/Voltage Measurement  PhasorSimulation=off  OutputType=Complex  PSBequivalent=0
  i : powerlib/Electrical Sources/Controlled Current Source  Initialize=on  Source_Type=AC  Amplitude=0  Phase=0  Frequency=0  Measurements=None
  +ve : PMIOPort  Port=1  Side=Right
  -ve : PMIOPort  Tag=PMCPort  Port=2  Side=Right
  wires:
  Voltage Measurement/1 -> Display/1
  Constant/1 -> i/1
  connections:
  Voltage Measurement/LConn1 -- 1/RConn1 -- +ve/RConn1
  Voltage Measurement/LConn2 -- -ve/RConn1 -- 2/RConn1 -- Diode/RConn1 -- i/LConn1
  2/LConn1 -- 1/LConn1 -- Diode/LConn1 -- i/RConn1

== system improved_z_source_inverterwithpv/Subsystem/PV 4 ==
  1 : powerlib/Elements/Series RLC Branch  LConnTagsString=__new0  RConnTagsString=__new0  BranchType=R  Resistance=0.001  Inductance=1e-3  SetiL0=off  InitialCurrent=0  Capacitance=1e-6  Setx0=off  InitialVoltage=0  Measurements=None
  2 : powerlib/Elements/Series RLC Branch  LConnTagsString=__new0  RConnTagsString=__new0  BranchType=R  Resistance=10000  Inductance=1e-3  SetiL0=off  InitialCurrent=0  Capacitance=1e-6  Setx0=off  InitialVoltage=0  Measurements=None
  Constant : Constant  Value=80
  Diode : powerlib/Power Electronics/Diode  Ron=0.001  Lon=0  Vf=20  IC=0  UseSnubber=off  Rs=500  Cs=250e-9  Measurements=off
  Display : Display
  Voltage Measurement : powerlib/Measurements/Voltage Measurement  PhasorSimulation=off  OutputType=Complex  PSBequivalent=0
  i : powerlib/Electrical Sources/Controlled Current Source  Initialize=on  Source_Type=AC  Amplitude=0  Phase=0  Frequency=0  Measurements=None
  +ve : PMIOPort  Port=1  Side=Right
  -ve : PMIOPort  Tag=PMCPort  Port=2  Side=Right
  wires:
  Constant/1 -> i/1
  Voltage Measurement/1 -> Display/1
  connections:
  i/RConn1 -- Diode/LConn1 -- 1/LConn1 -- 2/LConn1
  i/LConn1 -- Diode/RConn1 -- 2/RConn1 -- -ve/RConn1 -- Voltage Measurement/LConn2
  +ve/RConn1 -- 1/RConn1 -- Voltage Measurement/LConn1

== system improved_z_source_inverterwithpv/Subsystem/PV 5 ==
  1 : powerlib/Elements/Series RLC Branch  LConnTagsString=__new0  RConnTagsString=__new0  BranchType=R  Resistance=0.001  Inductance=1e-3  SetiL0=off  InitialCurrent=0  Capacitance=1e-6  Setx0=off  InitialVoltage=0  Measurements=None
  2 : powerlib/Elements/Series RLC Branch  LConnTagsString=__new0  RConnTagsString=__new0  BranchType=R  Resistance=10000  Inductance=1e-3  SetiL0=off  InitialCurrent=0  Capacitance=1e-6  Setx0=off  InitialVoltage=0  Measurements=None
  Constant : Constant  Value=80
  Diode : powerlib/Power Electronics/Diode  Ron=0.001  Lon=0  Vf=20  IC=0  UseSnubber=off  Rs=500  Cs=250e-9  Measurements=off
  Display : Display
  Voltage Measurement : powerlib/Measurements/Voltage Measurement  PhasorSimulation=off  OutputType=Complex  PSBequivalent=0
  i : powerlib/Electrical Sources/Controlled Current Source  Initialize=on  Source_Type=AC  Amplitude=0  Phase=0  Frequency=0  Measurements=None
  +ve : PMIOPort  Port=1  Side=Right
  -ve : PMIOPort  Tag=PMCPort  Port=2  Side=Right
  wires:
  Voltage Measurement/1 -> Display/1
  Constant/1 -> i/1
  connections:
  Voltage Measurement/LConn1 -- 1/RConn1 -- +ve/RConn1
  Voltage Measurement/LConn2 -- -ve/RConn1 -- 2/RConn1 -- Diode/RConn1 -- i/LConn1
  2/LConn1 -- 1/LConn1 -- Diode/LConn1 -- i/RConn1

== system improved_z_source_inverterwithpv/Subsystem/PV 6 ==
  1 : powerlib/Elements/Series RLC Branch  LConnTagsString=__new0  RConnTagsString=__new0  BranchType=R  Resistance=0.001  Inductance=1e-3  SetiL0=off  InitialCurrent=0  Capacitance=1e-6  Setx0=off  InitialVoltage=0  Measurements=None
  2 : powerlib/Elements/Series RLC Branch  LConnTagsString=__new0  RConnTagsString=__new0  BranchType=R  Resistance=10000  Inductance=1e-3  SetiL0=off  InitialCurrent=0  Capacitance=1e-6  Setx0=off  InitialVoltage=0  Measurements=None
  Constant : Constant  Value=80
  Diode : powerlib/Power Electronics/Diode  Ron=0.001  Lon=0  Vf=20  IC=0  UseSnubber=off  Rs=500  Cs=250e-9  Measurements=off
  Display : Display
  Voltage Measurement : powerlib/Measurements/Voltage Measurement  PhasorSimulation=off  OutputType=Complex  PSBequivalent=0
  i : powerlib/Electrical Sources/Controlled Current Source  Initialize=on  Source_Type=AC  Amplitude=0  Phase=0  Frequency=0  Measurements=None
  +ve : PMIOPort  Port=1  Side=Right
  -ve : PMIOPort  Tag=PMCPort  Port=2  Side=Right
  wires:
  Constant/1 -> i/1
  Voltage Measurement/1 -> Display/1
  connections:
  i/RConn1 -- Diode/LConn1 -- 1/LConn1 -- 2/LConn1
  i/LConn1 -- Diode/RConn1 -- 2/RConn1 -- -ve/RConn1 -- Voltage Measurement/LConn2
  +ve/RConn1 -- 1/RConn1 -- Voltage Measurement/LConn1

== system improved_z_source_inverterwithpv/Subsystem/PV 7 ==
  1 : powerlib/Elements/Series RLC Branch  LConnTagsString=__new0  RConnTagsString=__new0  BranchType=R  Resistance=0.001  Inductance=1e-3  SetiL0=off  InitialCurrent=0  Capacitance=1e-6  Setx0=off  InitialVoltage=0  Measurements=None
  2 : powerlib/Elements/Series RLC Branch  LConnTagsString=__new0  RConnTagsString=__new0  BranchType=R  Resistance=10000  Inductance=1e-3  SetiL0=off  InitialCurrent=0  Capacitance=1e-6  Setx0=off  InitialVoltage=0  Measurements=None
  Constant : Constant  Value=80
  Diode : powerlib/Power Electronics/Diode  Ron=0.001  Lon=0  Vf=20  IC=0  UseSnubber=off  Rs=500  Cs=250e-9  Measurements=off
  Display : Display
  Voltage Measurement : powerlib/Measurements/Voltage Measurement  PhasorSimulation=off  OutputType=Complex  PSBequivalent=0
  i : powerlib/Electrical Sources/Controlled Current Source  Initialize=on  Source_Type=AC  Amplitude=0  Phase=0  Frequency=0  Measurements=None
  +ve : PMIOPort  Port=1  Side=Right
  -ve : PMIOPort  Tag=PMCPort  Port=2  Side=Right
  wires:
  Voltage Measurement/1 -> Display/1
  Constant/1 -> i/1
  connections:
  Voltage Measurement/LConn1 -- 1/RConn1 -- +ve/RConn1
  Voltage Measurement/LConn2 -- -ve/RConn1 -- 2/RConn1 -- Diode/RConn1 -- i/LConn1
  2/LConn1 -- 1/LConn1 -- Diode/LConn1 -- i/RConn1

== system improved_z_source_inverterwithpv/Subsystem/PV 8 ==
  1 : powerlib/Elements/Series RLC Branch  LConnTagsString=__new0  RConnTagsString=__new0  BranchType=R  Resistance=0.001  Inductance=1e-3  SetiL0=off  InitialCurrent=0  Capacitance=1e-6  Setx0=off  InitialVoltage=0  Measurements=None
  2 : powerlib/Elements/Series RLC Branch  LConnTagsString=__new0  RConnTagsString=__new0  BranchType=R  Resistance=10000  Inductance=1e-3  SetiL0=off  InitialCurrent=0  Capacitance=1e-6  Setx0=off  InitialVoltage=0  Measurements=None
  Constant : Constant  Value=80
  Diode : powerlib/Power Electronics/Diode  Ron=0.001  Lon=0  Vf=20  IC=0  UseSnubber=off  Rs=500  Cs=250e-9  Measurements=off
  Display : Display
  Voltage Measurement : powerlib/Measurements/Voltage Measurement  PhasorSimulation=off  OutputType=Complex  PSBequivalent=0
  i : powerlib/Electrical Sources/Controlled Current Source  Initialize=on  Source_Type=AC  Amplitude=0  Phase=0  Frequency=0  Measurements=None
  +ve : PMIOPort  Port=1  Side=Right
  -ve : PMIOPort  Tag=PMCPort  Port=2  Side=Right
  wires:
  Constant/1 -> i/1
  Voltage Measurement/1 -> Display/1
  connections:
  i/RConn1 -- Diode/LConn1 -- 1/LConn1 -- 2/LConn1
  i/LConn1 -- Diode/RConn1 -- 2/RConn1 -- -ve/RConn1 -- Voltage Measurement/LConn2
  +ve/RConn1 -- 1/RConn1 -- Voltage Measurement/LConn1

== system improved_z_source_inverterwithpv/Subsystem/PV 9 ==
  1 : powerlib/Elements/Series RLC Branch  LConnTagsString=__new0  RConnTagsString=__new0  BranchType=R  Resistance=0.001  Inductance=1e-3  SetiL0=off  InitialCurrent=0  Capacitance=1e-6  Setx0=off  InitialVoltage=0  Measurements=None
  2 : powerlib/Elements/Series RLC Branch  LConnTagsString=__new0  RConnTagsString=__new0  BranchType=R  Resistance=10000  Inductance=1e-3  SetiL0=off  InitialCurrent=0  Capacitance=1e-6  Setx0=off  InitialVoltage=0  Measurements=None
  Constant : Constant  Value=80
  Diode : powerlib/Power Electronics/Diode  Ron=0.001  Lon=0  Vf=20  IC=0  UseSnubber=off  Rs=500  Cs=250e-9  Measurements=off
  Display : Display
  Voltage Measurement : powerlib/Measurements/Voltage Measurement  PhasorSimulation=off  OutputType=Complex  PSBequivalent=0
  i : powerlib/Electrical Sources/Controlled Current Source  Initialize=on  Source_Type=AC  Amplitude=0  Phase=0  Frequency=0  Measurements=None
  +ve : PMIOPort  Port=1  Side=Right
  -ve : PMIOPort  Tag=PMCPort  Port=2  Side=Right
  wires:
  Voltage Measurement/1 -> Display/1
  Constant/1 -> i/1
  connections:
  Voltage Measurement/LConn1 -- 1/RConn1 -- +ve/RConn1
  Voltage Measurement/LConn2 -- -ve/RConn1 -- 2/RConn1 -- Diode/RConn1 -- i/LConn1
  2/LConn1 -- 1/LConn1 -- Diode/LConn1 -- i/RConn1
